simulink model "pideffort"  (R2020a)
settings: Solver=VariableStepAuto  StartTime=0.0  StopTime=1e5  FixedStep=44.2247  RelTol=1e-3
libraries: cstblocks x2
settings Model: Creator=jose  LastModifiedBy=jose

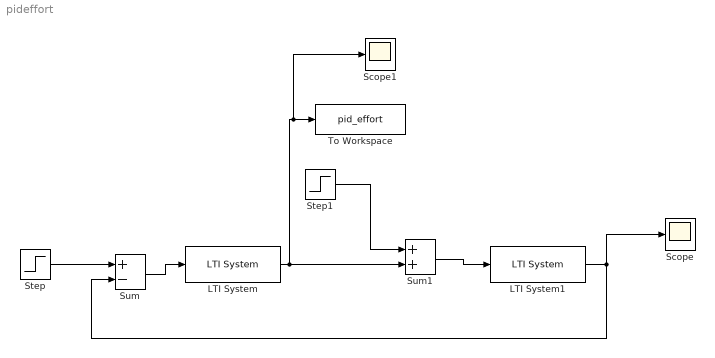
== system pideffort ==
  LTI System : cstblocks/LTI System  sys=Cd_dr  IC=[]
  LTI System1 : cstblocks/LTI System  sys=Gd_d  IC=[]
  Scope : Scope
  Scope1 : Scope
  Step : Step  Time=0  After=0  SampleTime=0
  Step1 : Step  Before=0.25  After=0.25  SampleTime=0
  Sum : Sum  Inputs=+-  InputSameDT=on  SaturateOnIntegerOverflow=on  OutDataTypeStr=Inherit: Same as first input
  Sum1 : Sum  InputSameDT=on  SaturateOnIntegerOverflow=on  OutDataTypeStr=Inherit: Same as first input
  To Workspace : ToWorkspace  VariableName=pid_effort  SaveFormat=Timeseries  SampleTime=-1
  wires:
  Step1/1 -> Sum1/1
  Sum/1 -> LTI System/1
  Step/1 -> Sum/1
  LTI System1/1 -> Scope/1, Sum/2
  Sum1/1 -> LTI System1/1
  LTI System/1 -> Sum1/2, Scope1/1, To Workspace/1
